simulink model "temperaturesensing"  (R2022a)
settings: Solver=VariableStepAuto  StartTime=0.0  StopTime=10.0  RelTol=1e-3
undefined symbols (not defined in the file): r
libraries: simulink x3, simulink_extras x1
settings Model: Creator=wel  LastModifiedBy=wel

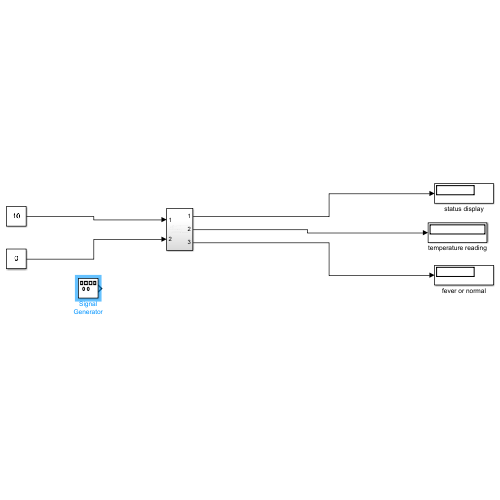
[thumbnail: Simulink's stored preview of the top-level diagram]
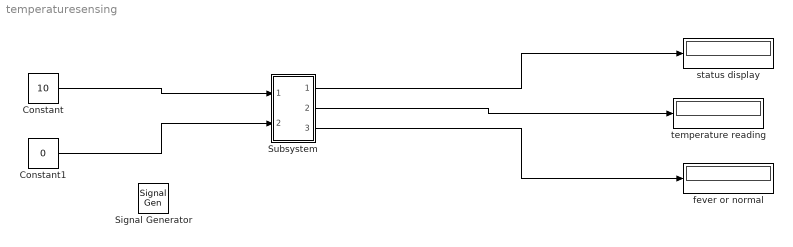
== system temperaturesensing ==
  Constant : Constant  Value=10  VectorParams1D=off
  Constant1 : Constant  Value=0
  Signal Generator : SignalGenerator  Units=rad/sec
  Subsystem : Subsystem
  fever or normal : Display
  status display : Display
  temperature reading : Display
  wires:
  Subsystem/1(Out2) -> status display/1
  Constant1/1 -> Subsystem/2(In2)
  Subsystem/3(Out3) -> fever or normal/1
  Constant/1 -> Subsystem/1(In1)
  Subsystem/2(Out1) -> temperature reading/1

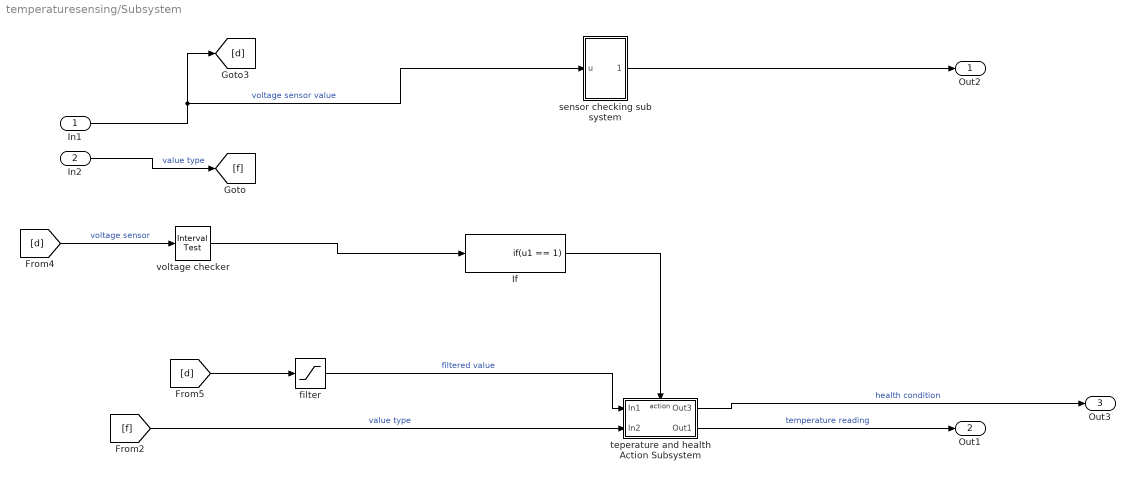
== system temperaturesensing/Subsystem ==
  In1 : Inport
  In2 : Inport  Port=2
  If : If  IfExpression=u1 == 1  ShowElse=off
  filter : Saturate  UpperLimit=15  LowerLimit=0
  sensor checking sub system : Subsystem
  teperature and health Action Subsystem : Subsystem  TreatAsAtomicUnit=on
  voltage checker : simulink/Logic and Bit Operations/Interval Test  IntervalClosedRight=on  uplimit=15  IntervalClosedLeft=on  lowlimit=0  OutDataTypeStr=boolean
  Out2 : Outport
  Out1 : Outport  Port=2
  Out3 : Outport  Port=3
  wires:
  In1/1 -> sensor checking sub system/1(u), [d]  "voltage sensor value"
  [d] -> voltage checker/1  "voltage sensor"
  voltage checker/1 -> If/1
  [d] -> filter/1
  filter/1 -> teperature and health Action Subsystem/1(In1)  "filtered value"
  If/1 -> teperature and health Action Subsystem/Action
  In2/1 -> [f]  "value type"
  [f] -> teperature and health Action Subsystem/2(In2)  "value type"
  teperature and health Action Subsystem/2(Out1) -> Out1/1  "temperature reading"
  teperature and health Action Subsystem/1(Out3) -> Out3/1  "health condition"
  sensor checking sub system/1(Out1) -> Out2/1

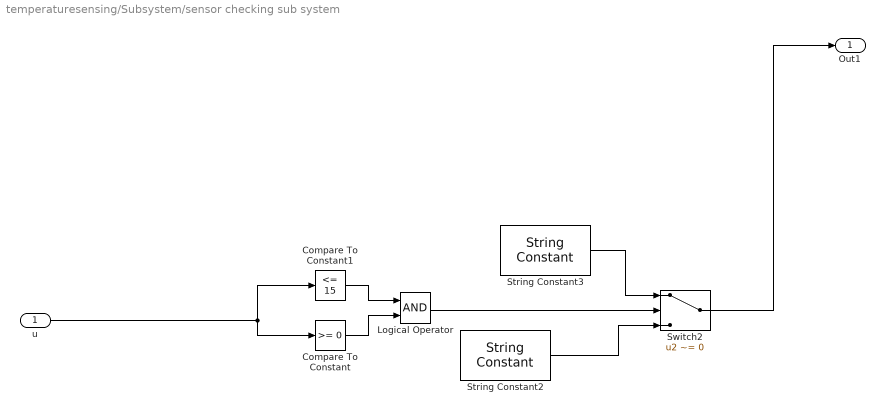
== system temperaturesensing/Subsystem/sensor checking sub system ==
  u : Inport
  Compare To Constant : simulink/Logic and Bit Operations/Compare To Constant  relop=>=  const=0  OutDataTypeStr=boolean
  Compare To Constant1 : simulink/Logic and Bit Operations/Compare To Constant  relop=<=  const=15  OutDataTypeStr=boolean
  Logical Operator : Logic  AllPortsSameDT=off  OutDataTypeStr=boolean
  String Constant2 : StringConstant  String=n
  String Constant3 : StringConstant  String=m
  Switch2 : Switch  Criteria=u2 ~= 0  Threshold=15  SaturateOnIntegerOverflow=off  InputSameDT=off
  Out1 : Outport
  wires:
  String Constant2/1 -> Switch2/3
  String Constant3/1 -> Switch2/1
  Compare To Constant/1 -> Logical Operator/2
  u/1 -> Compare To Constant/1, Compare To Constant1/1
  Logical Operator/1 -> Switch2/2
  Compare To Constant1/1 -> Logical Operator/1
  Switch2/1 -> Out1/1

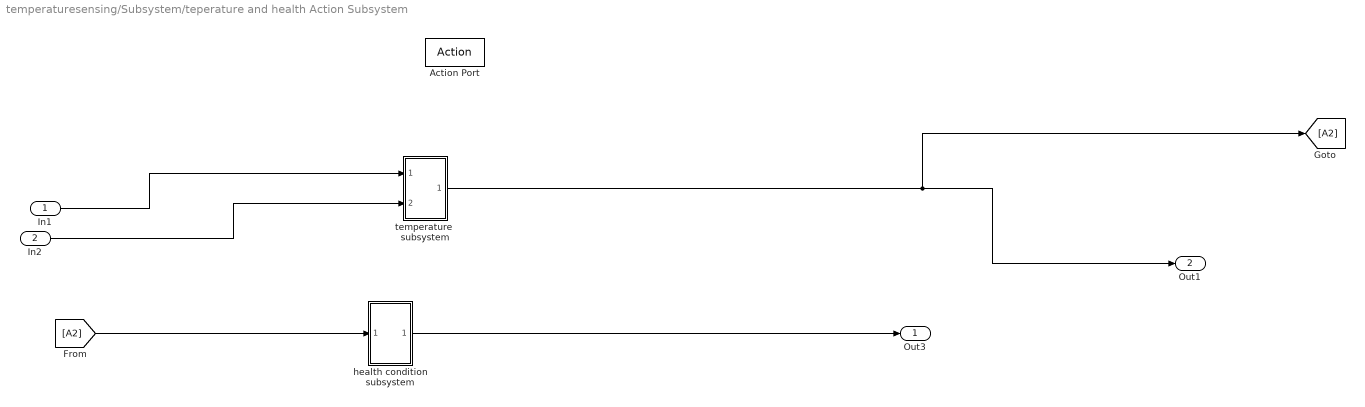
== system temperaturesensing/Subsystem/teperature and health Action Subsystem ==
  In1 : Inport
  In2 : Inport  Port=2
  Action Port : ActionPort
  health condition subsystem : Subsystem
  temperature  subsystem : Subsystem
  Out3 : Outport
  Out1 : Outport  Port=2
  wires:
  In1/1 -> temperature  subsystem/1(In1)
  In2/1 -> temperature  subsystem/2(In2)
  temperature  subsystem/1(Out1) -> [A2], Out1/1
  [A2] -> health condition subsystem/1(In1)
  health condition subsystem/1(Out1) -> Out3/1

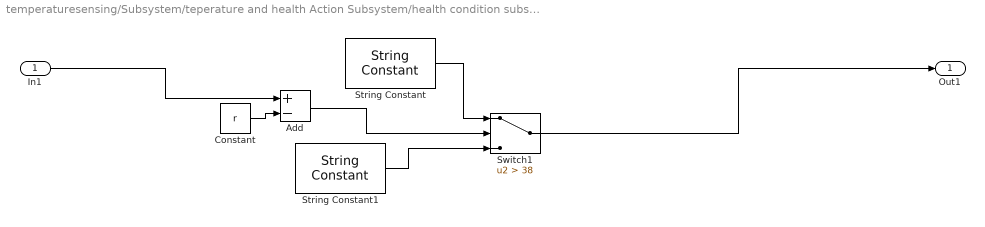
== system temperaturesensing/Subsystem/teperature and health Action Subsystem/health condition subsystem ==
  In1 : Inport
  Add : Sum  Inputs=+-
  Constant : Constant  Value=r
  String Constant : StringConstant  String="\"fever\""
  String Constant1 : StringConstant  String="\"normal\""
  Switch1 : Switch  Criteria=u2 > Threshold  Threshold=38  SaturateOnIntegerOverflow=off  InputSameDT=off
  Out1 : Outport
  wires:
  Add/1 -> Switch1/2
  String Constant/1 -> Switch1/1
  String Constant1/1 -> Switch1/3
  Constant/1 -> Add/2
  In1/1 -> Add/1
  Switch1/1 -> Out1/1

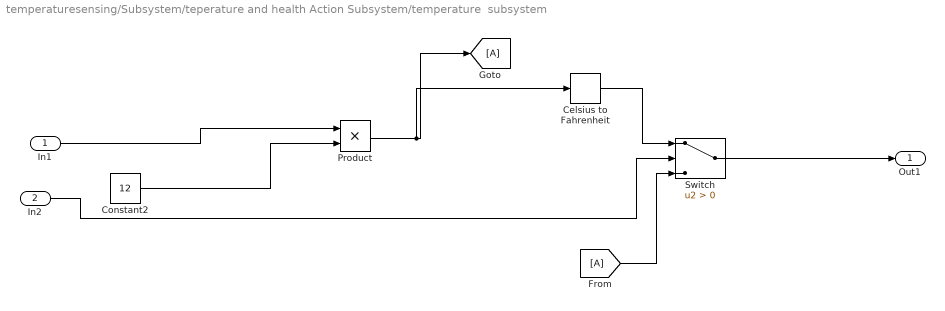
== system temperaturesensing/Subsystem/teperature and health Action Subsystem/temperature  subsystem ==
  In1 : Inport
  In2 : Inport  Port=2
  Celsius to Fahrenheit : simulink_extras/Transformations/Celsius to Fahrenheit
      settings: SourceProductBaseCode=SL
  Constant2 : Constant  Value=12
  From : From
  Goto : Goto
  Product : Product
  Switch : Switch  Criteria=u2 > Threshold  SaturateOnIntegerOverflow=off  InputSameDT=off
  Out1 : Outport
  wires:
  Celsius to Fahrenheit/1 -> Switch/1
  Switch/1 -> Out1/1
  In2/1 -> Switch/2
  From/1 -> Switch/3
  In1/1 -> Product/1
  Constant2/1 -> Product/2
  Product/1 -> Celsius to Fahrenheit/1, Goto/1
